simulink model "simulador"  (R2020a)
settings: Solver=VariableStepAuto  StartTime=0.0  StopTime=200  RelTol=1e-3
InitFcn:
  | initialize
values from neighbouring files (symbols this model uses):
  d_min = 10    [initialize.m]
  fault_d = 200    [initialize.m]
  K_lin = 0.05    [initialize.m]
  P_ego_init = 0    [initialize.m]
  P_lead_init = P_ego_init + 30    (= 30)    [initialize.m]
  t_gap = 1.5    [initialize.m]
  tau_lin = 81.1    [initialize.m]
  V_ego_init = 110/3.6    (= 30.5555555556)    [initialize.m]
  V_lead_init = 110/3.6    (= 30.5555555556)    [initialize.m]
libraries: mpcadaslib x1
settings Model: Creator=derpb  LastModifiedBy=derpb
settings DataIOCC: ReturnWorkspaceOutputs=off
settings DebuggingCC: ArithmeticOperatorsInVariantConditions=warning
settings SFSimCC: CustomCodeUndefinedFunction=UseInterfaceOnly

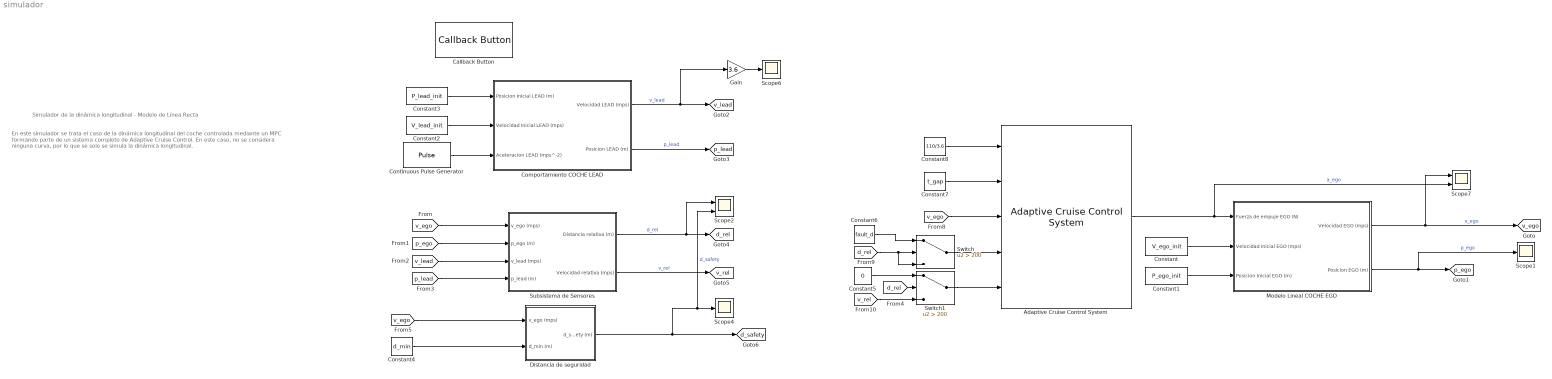
== system simulador ==
  note: En este simulador se trata el caso de la dinámica longitudinal del coche controlada mediante un MPC
      | formando parte de un sistema completo de Adaptive Cruise Control. En este caso, no se considera ninguna
      | curva, por lo que se solo se simula la dinámica longitudinal.
  note: Simulador de la dinámica longitudinal - Modelo de Línea Recta
  Adaptive Cruise Control System : mpcadaslib/Adaptive Cruise Control System  EgoModel=tf(0.05,[81.1,1])  InitialEgoVelocity=110/3.6  DefaultSpacing=10  MaxVelocity=120/3.6  MinAcceleration=-3000  amin_ext=off  MaxAcceleration=2000  amax_ext=off  Ts=0.1  PredictionHorizon=30  ControllerBehavior=0.700  suboptimal=off  maxiter=10  datatypeopt=double  optmode=off  trackmode=off
  Callback Button : CallbackButton  ButtonText=INICIALIZACION
      settings: ClickFcn=initialize
  Comportamiento COCHE LEAD : Subsystem
  Constant : Constant  Value=V_ego_init
  Constant1 : Constant  Value=P_ego_init
  Constant2 : Constant  Value=V_lead_init
  Constant3 : Constant  Value=P_lead_init
  Constant4 : Constant  Value=d_min
  Constant5 : Constant  Value=0
  Constant6 : Constant  Value=fault_d
  Constant7 : Constant  Value=t_gap
  Constant8 : Constant  Value=110/3.6
  Continuous Pulse Generator : DiscretePulseGenerator  PulseType=Time based  Amplitude=-2  Period=50  PulseWidth=1/4  PhaseDelay=10
  Distancia de seguridad : Subsystem
  Gain : Gain  Gain=3.6
  Modelo Lineal COCHE EGO : Subsystem
  Scope1 : Scope
  Scope2 : Scope  NumInputPorts=2
  Scope4 : Scope
  Scope6 : Scope
  Scope7 : Scope  NumInputPorts=2
  Subsistema de Sensores : Subsystem
  Switch : Switch  Criteria=u2 > Threshold  Threshold=200
  Switch1 : Switch  Criteria=u2 > Threshold  Threshold=200
  tag scope: d_rel=global, d_safety=global, p_ego=global, p_lead=global, v_ego=global, v_lead=global, v_rel=global
  wires:
  Constant/1 -> Modelo Lineal COCHE EGO/2(Velocidad Inicial EGO (mps))
  Modelo Lineal COCHE EGO/1(Velocidad EGO (mps)) -> Scope7/1, [v_ego]  "v_ego"
  Modelo Lineal COCHE EGO/2(Posicion EGO (m)) -> Scope1/1, [p_ego]  "p_ego"
  Comportamiento COCHE LEAD/1(Velocidad LEAD (mps)) -> Gain/1, [v_lead]  "v_lead"
  Comportamiento COCHE LEAD/2(Posicion LEAD (m)) -> [p_lead]  "p_lead"
  Constant1/1 -> Modelo Lineal COCHE EGO/3(Posicion Inicial EGO (m))
  Constant2/1 -> Comportamiento COCHE LEAD/2(Velocidad Inicial LEAD (mps))
  Constant3/1 -> Comportamiento COCHE LEAD/1(Posicion Inicial LEAD (m))
  [v_ego] -> Subsistema de Sensores/1(v_ego (mps))
  [p_ego] -> Subsistema de Sensores/2(p_ego (m))
  [v_lead] -> Subsistema de Sensores/3(v_lead (mps))
  [p_lead] -> Subsistema de Sensores/4(p_lead (m))
  Subsistema de Sensores/1(Distancia relativa (m)) -> Scope2/1, [d_rel]  "d_rel"
  Subsistema de Sensores/2(Velocidad relativa (mps)) -> [v_rel]  "v_rel"
  Constant4/1 -> Distancia de seguridad/2(d_min (m))
  Distancia de seguridad/1(d_safety (m)) -> Scope2/2, Scope4/1, [d_safety]  "d_safety"
  [v_ego] -> Distancia de seguridad/1(v_ego (mps))
  Constant7/1 -> Adaptive Cruise Control System/2
  [v_ego] -> Adaptive Cruise Control System/3
  Constant8/1 -> Adaptive Cruise Control System/1
  Adaptive Cruise Control System/1 -> Scope7/2, Modelo Lineal COCHE EGO/1(Fuerza de empuje EGO (N))  "a_ego"
  Gain/1 -> Scope6/1
  Switch/1 -> Adaptive Cruise Control System/4
  [d_rel] -> Switch/3, Switch/2
  [v_rel] -> Switch1/3
  [d_rel] -> Switch1/2
  Constant5/1 -> Switch1/1
  Switch1/1 -> Adaptive Cruise Control System/5
  Constant6/1 -> Switch/1
  Continuous Pulse Generator/1 -> Comportamiento COCHE LEAD/3(Aceleracion LEAD (mps^-2))

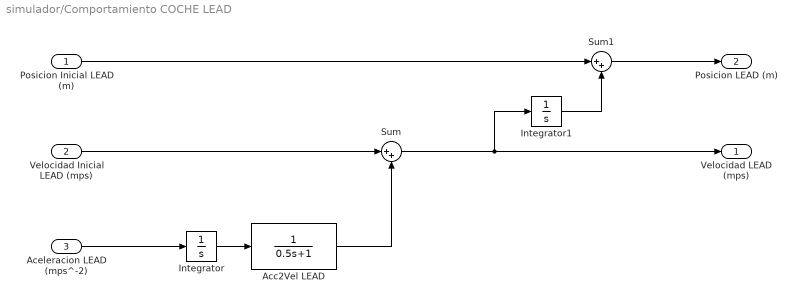
== system simulador/Comportamiento COCHE LEAD ==
  Posicion Inicial LEAD (m) : Inport
  Velocidad Inicial LEAD (mps) : Inport  Port=2
  Aceleracion LEAD (mps^-2) : Inport  Port=3
  Acc2Vel LEAD : TransferFcn  Denominator=[0.5 1]
  Integrator : Integrator
  Integrator1 : Integrator
  Sum : Sum  Inputs=|++
  Sum1 : Sum  Inputs=|++
  Velocidad LEAD (mps) : Outport  VectorParamsAs1DForOutWhenUnconnected=off
  Posicion LEAD (m) : Outport  Port=2  VectorParamsAs1DForOutWhenUnconnected=off
  wires:
  Integrator/1 -> Acc2Vel LEAD/1
  Aceleracion LEAD (mps^-2)/1 -> Integrator/1
  Velocidad Inicial LEAD (mps)/1 -> Sum/1
  Acc2Vel LEAD/1 -> Sum/2
  Sum/1 -> Integrator1/1, Velocidad LEAD (mps)/1
  Sum1/1 -> Posicion LEAD (m)/1
  Integrator1/1 -> Sum1/2
  Posicion Inicial LEAD (m)/1 -> Sum1/1

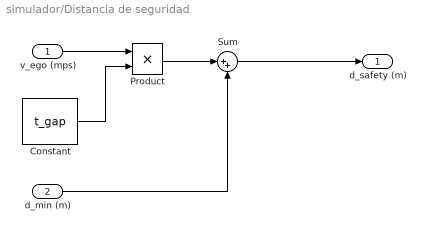
== system simulador/Distancia de seguridad ==
  v_ego (mps) : Inport
  d_min (m) : Inport  Port=2
  Constant : Constant  Value=t_gap
  Product : Product
  Sum : Sum  Inputs=|++
  d_safety (m) : Outport  VectorParamsAs1DForOutWhenUnconnected=off
  wires:
  v_ego (mps)/1 -> Product/1
  Constant/1 -> Product/2
  Product/1 -> Sum/1
  Sum/1 -> d_safety (m)/1
  d_min (m)/1 -> Sum/2

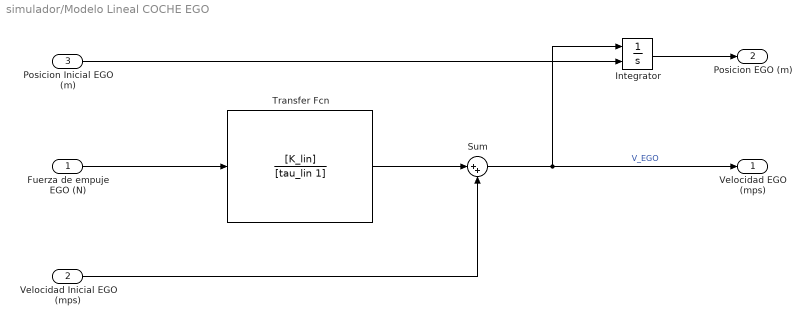
== system simulador/Modelo Lineal COCHE EGO ==
  Fuerza de empuje EGO (N) : Inport
  Velocidad Inicial EGO (mps) : Inport  Port=2
  Posicion Inicial EGO (m) : Inport  Port=3
  Integrator : Integrator  InitialConditionSource=external
  Sum : Sum  Inputs=|++
  Transfer Fcn : TransferFcn  Numerator=[K_lin]  Denominator=[tau_lin 1]
  Velocidad EGO (mps) : Outport  VectorParamsAs1DForOutWhenUnconnected=off
  Posicion EGO (m) : Outport  Port=2  VectorParamsAs1DForOutWhenUnconnected=off
  wires:
  Transfer Fcn/1 -> Sum/1
  Sum/1 -> Integrator/1, Velocidad EGO (mps)/1  "V_EGO"
  Velocidad Inicial EGO (mps)/1 -> Sum/2
  Posicion Inicial EGO (m)/1 -> Integrator/2
  Integrator/1 -> Posicion EGO (m)/1
  Fuerza de empuje EGO (N)/1 -> Transfer Fcn/1

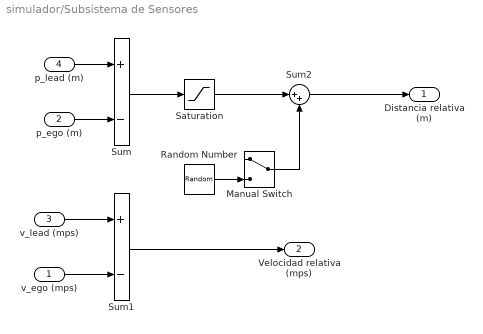
== system simulador/Subsistema de Sensores ==
  v_ego (mps) : Inport
  p_ego (m) : Inport  Port=2
  v_lead (mps) : Inport  Port=3
  p_lead (m) : Inport  Port=4
  Manual Switch : ManualSwitch
  Random Number : RandomNumber  Variance=0.06  SampleTime=0.1
  Saturation : Saturate  UpperLimit=fault_d  LowerLimit=0
  Sum : Sum  Inputs=+-
  Sum1 : Sum  Inputs=+-
  Sum2 : Sum  Inputs=|++
  Distancia relativa (m) : Outport  VectorParamsAs1DForOutWhenUnconnected=off
  Velocidad relativa (mps) : Outport  Port=2  VectorParamsAs1DForOutWhenUnconnected=off
  wires:
  Sum/1 -> Saturation/1
  p_lead (m)/1 -> Sum/1
  p_ego (m)/1 -> Sum/2
  v_lead (mps)/1 -> Sum1/1
  v_ego (mps)/1 -> Sum1/2
  Sum1/1 -> Velocidad relativa (mps)/1
  Saturation/1 -> Sum2/1
  Sum2/1 -> Distancia relativa (m)/1
  Random Number/1 -> Manual Switch/2
  Manual Switch/1 -> Sum2/2
